simulink model "arm_sim_lin"  (Simulink 7.7)
settings: Solver=ode45  StartTime=0.0  StopTime=100  RelTol=1e-3
settings Model: Creator=beard  LastModifiedBy=beard
settings OptimizationCC: InitFltsAndDblsToZero=on
settings DebuggingCC: StrictBusMsg=Warning

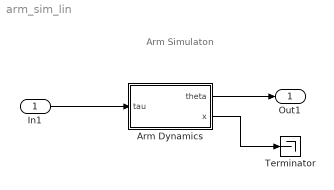
== system arm_sim_lin ==
  note: Arm Simulaton
  In1 : Inport
  Arm Dynamics : Subsystem
  Terminator : Terminator
  Out1 : Outport
  wires:
  Arm Dynamics/1(theta) -> Out1/1
  Arm Dynamics/2(x) -> Terminator/1
  In1/1 -> Arm Dynamics/1(tau)

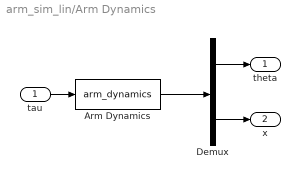
== system arm_sim_lin/Arm Dynamics ==
  tau : Inport
  Arm Dynamics : S-Function  FunctionName=arm_dynamics  Parameters=AP  EnableBusSupport=off
  Demux : Demux  Outputs=[1;2]
  theta : Outport
  x : Outport  Port=2
  wires:
  tau/1 -> Arm Dynamics/1
  Arm Dynamics/1 -> Demux/1
  Demux/1 -> theta/1
  Demux/2 -> x/1
